simulink model "JABS"  (R2018b)
settings: Solver=FixedStepDiscrete  StartTime=0.0  StopTime=10.0  FixedStep=0.01  RelTol=1e-3
(part 1 of 2)
settings Model: Creator=gaohang  LastModifiedBy=gaohang
settings OptimizationCC: BlockReduction=off  DefaultParameterBehavior=Inlined  UseDivisionForNetSlopeComputation=on  UseFloatMulNetSlope=on  DefaultUnderspecifiedDataType=single  UseSpecifiedMinMax=on  InlineInvariantSignals=on  PassReuseOutputArgsAs=Individual arguments  ZeroExternalMemoryAtStartup=off  ZeroInternalMemoryAtStartup=off  LifeSpan=inf  OptimizeBlockOrder=speed  DifferentSizesBufferReuse=on
settings DebuggingCC: SignalInfNanChecking=error  ReadBeforeWriteMsg=EnableAllAsError  WriteAfterWriteMsg=EnableAllAsError  WriteAfterReadMsg=EnableAllAsError  IntegerOverflowMsg=error  ParameterTunabilityLossMsg=error  UniqueDataStoreMsg=error  NonBusSignalsTreatedAsBus=error  IntegerSaturationMsg=error
settings ModelReferenceCC: UpdateModelReferenceTargets=IfOutOfDate
settings SFSimCC: SFSimEcho=off  CompileTimeRecursionLimit=0  MATLABDynamicMemAlloc=off
settings RTWCC: SystemTargetFile=autosar.tlc  GenCodeOnly=on  TemplateMakefile=ert_default_tmf  Description=AUTOSAR  GenerateReport=on  BuildConfiguration=Faster Runs  IncludeHyperlinkInReport=on  LaunchReport=on  GenerateTraceInfo=on  GenerateTraceReport=on  GenerateTraceReportSl=on  GenerateTraceReportSf=on  GenerateTraceReportEml=on  GenerateCodeMetricsReport=on
settings CodeAppCC: ForceParamTrailComments=on  IgnoreCustomStorageClasses=off  OperatorAnnotations=on  SimulinkDataObjDesc=on  SFDataObjDesc=on  MATLABFcnDesc=on  InsertBlockDesc=on  StateflowObjectComments=on  EnableCustomComments=on  ReqsInCode=on
settings STFCustomTargetCC: TargetLangStandard=C99 (ISO)  UtilityFuncGeneration=Shared location  MultiwordLength=256  ParMdlRefBuildCompliant=on  CompOptLevelCompliant=on  IncludeMdlTerminateFcn=off  CombineOutputUpdateFcns=on  CombineSignalStateStructs=on  SuppressErrorStatus=on  ERTCustomFileBanners=on  SupportNonFinite=off  SupportComplex=off  SupportContinuousTime=off  SupportNonInlinedSFcns=off  RemoveResetFunc=on  ParenthesesLevel=Maximum  CastingMode=Standards  MATLABClassNameForMDSCustomization=Simulink.SoftwareTarget.ERTCustomization  AutosarCompliant=on  UseToolchainInfoCompliant=on  GenerateSharedConstants=off  LookupTableObjectStructAxisOrder=2,1,3,4,...  LUTObjectStructOrderEvenSpacing=Size,Table,Breakpoints  SystemTargetFile=autosar.tlc
settings ERTTargetCC: TargetLangStandard=C99 (ISO)  UtilityFuncGeneration=Shared location  ConcurrentExecutionCompliant=off  IncludeMdlTerminateFcn=off  CombineSignalStateStructs=on  SuppressErrorStatus=on  SupportNonFinite=off  SupportComplex=off  ParenthesesLevel=Maximum  CastingMode=Standards  ModelStepFunctionPrototypeControlCompliant=off  CPPClassGenCompliant=off  AutosarCompliant=on  GenerateSharedConstants=off  LookupTableObjectStructAxisOrder=2,1,3,4,...  LUTObjectStructOrderEvenSpacing=Size,Table,Breakpoints  GenerateASAP2=on  InlinedParameterPlacement=NonHierarchical  ERTCustomFileTemplate=example_file_process.tlc  EnableSignedLeftShifts=off  EnableSignedRightShifts=off

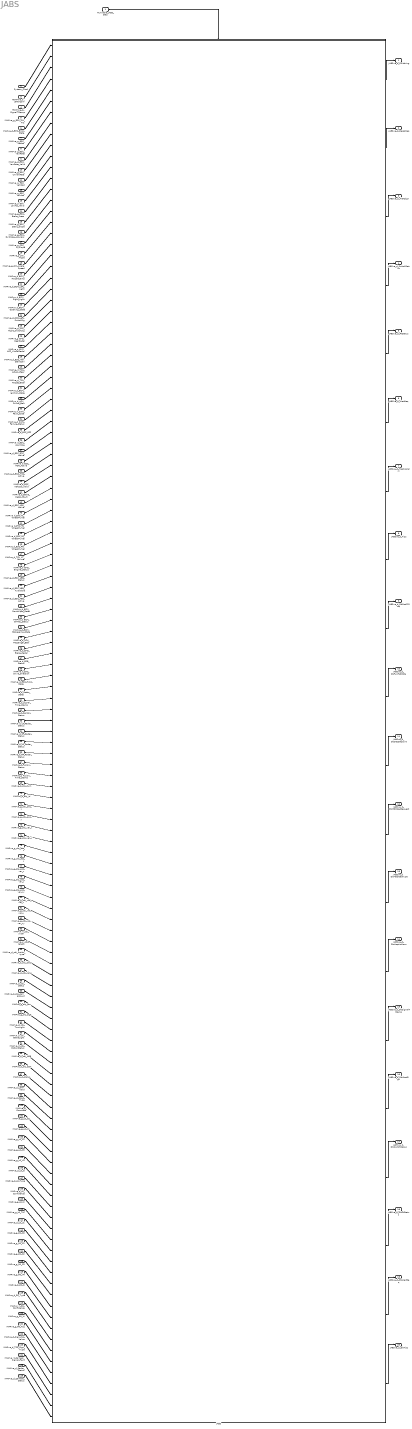
== system JABS ==
  Runnable_JABS_Step : Inport  SampleTime=0.01  OutputFunctionCall=on
  System_Clock : Inport  Port=2
  FDMMve_d_JaFcnConf : Inport  Port=3
  FDMMve_d_SignalTStamp : Inport  Port=4
  IMAPve_g_EPS_SW_Trq : Inport  Port=5
  IMAPve_d_EPS_Error_State : Inport  Port=6
  IMAPve_g_ESC_LatAcc : Inport  Port=7
  IMAPve_g_ESC_YawRate : Inport  Port=8
  IMAPve_d_ESC_YawRate_Valid : Inport  Port=9
  IMAPve_g_ESC_UnYawRate : Inport  Port=10
  IMAPve_g_ESC_VehSpd : Inport  Port=11
  IMAPve_g_ESC_LonAcc : Inport  Port=12
  IMAPve_d_ESC_LonAcc_Valid : Inport  Port=13
  IMAPve_g_ESC_Brake_Press : Inport  Port=14
  IMAPve_g_ESC_Static_Slope : Inport  Port=15
  IMAPve_g_ESC_DySlope_Accuracy : Inport  Port=16
  IMAPve_g_ESC_DySlope : Inport  Port=17
  IMAPve_g_SW_Angle : Inport  Port=18
  IMAPve_g_SW_Angle_Speed : Inport  Port=19
  IMAPve_d_BCM_HazardLamp : Inport  Port=20
  IMAPve_d_BCM_Left_Light : Inport  Port=21
  IMAPve_d_BCM_Right_Light : Inport  Port=22
  IMAPve_d_BCM_Opening_State : Inport  Port=23
  IMAPve_d_SCC_Left_SwitchSig : Inport  Port=24
  IMAPve_d_SCC_Right_SwitchSig : Inport  Port=25
  IMAPve_g_EMS_RealPedal : Inport  Port=26
  IMAPve_g_EMS_ACC_VirtualPedal : Inport  Port=27
  IMAPve_d_ESC_Veh_Standstill : Inport  Port=28
  IMAPve_d_TCU_Actual_Gear : Inport  Port=29
  IMAPve_d_TCU_Target_Gear : Inport  Port=30
  IMAPve_d_BCM_Ignition_State : Inport  Port=31
  IMAPve_d_ACU_Driver_Belt : Inport  Port=32
  IMAPve_d_SWS_Fault_Code : Inport  Port=33
  IMAPve_d_SWS_Failure_Status : Inport  Port=34
  IMAPve_d_ESC_OFF : Inport  Port=35
  IMAPve_d_ESC_AlarmSig : Inport  Port=36
  IMAPve_d_ESC_ESC_Active : Inport  Port=37
  IMAPve_d_ESC_MSR_Active : Inport  Port=38
  IMAPve_d_ESC_TCS_Active : Inport  Port=39
  IMAPve_d_ESC_VehSpd_Valid : Inport  Port=40
  IMAPve_d_Brake_Pedal_Fault : Inport  Port=41
  IMAPve_d_ESC_ABS_Active : Inport  Port=42
  IMAPve_d_ESC_FL_WheelPulVal : Inport  Port=43
  IMAPve_d_ESC_FR_WheelPulVal : Inport  Port=44
  IMAPve_d_ESC_RL_WheelPulVal : Inport  Port=45
  IMAPve_d_ESC_RR_WheelPulVal : Inport  Port=46
  IMAPve_d_TCU_AT_Failure : Inport  Port=47
  IMAPve_d_EMS_Engine_Status : Inport  Port=48
  IMAPve_d_ESC_AEB_Status : Inport  Port=49
  IMAPve_d_ESC_AEB_Available : Inport  Port=50
  IMAPve_d_ESC_AEB_Active : Inport  Port=51
  IMAPve_d_BCM_FrontWiper_State : Inport  Port=52
  IMAPve_d_BCM_CHMSL_Status : Inport  Port=53
  IMAPve_d_BCM_BrakeLamp_State : Inport  Port=54
  IMAPve_d_ACU_Passenger_Belt : Inport  Port=55
  IMAPve_d_EMS_Brake_Pedal : Inport  Port=56
  IMAPve_d_EPB_Status : Inport  Port=57
  IMAPve_d_ESC_Drive_Direction : Inport  Port=58
  IMAPve_d_ESC_Hold_State : Inport  Port=59
  IMAPve_d_Radar_State : Inport  Port=60
  IMAPve_d_Signal_Time_Stamp : Inport  Port=61
  IMAPve_d_Sensor_Status : Inport  Port=62
  IMAPve_d_LF_Radar_Status : Inport  Port=63
  IMAPve_d_RF_Radar_Status : Inport  Port=64
  IMAPve_d_LR_Radar_Status : Inport  Port=65
  IMAPve_d_RR_Radar_Status : Inport  Port=66
  IMAPve_d_Fusion_Status : Inport  Port=67
  IMAPve_g_Fusion_Time_Stamp : Inport  Port=68
  IMAPve_d_obj_Num : Inport  Port=69
  IMAPva_d_obj_id : Inport  Port=70
  IMAPva_g_obj_pos_x : Inport  Port=71
  IMAPva_g_obj_pos_y : Inport  Port=72
  IMAPva_g_obj_vel_x : Inport  Port=73
  IMAPva_g_obj_vel_y : Inport  Port=74
  IMAPva_g_obj_acc_x : Inport  Port=75
  IMAPva_g_obj_acc_y : Inport  Port=76
  IMAPva_g_obj_pos_var_x : Inport  Port=77
  IMAPva_g_obj_pos_var_y : Inport  Port=78
  IMAPva_g_obj_pos_var_xy : Inport  Port=79
  IMAPva_g_obj_vel_var_x : Inport  Port=80
  IMAPva_g_obj_vel_var_y : Inport  Port=81
  IMAPva_g_obj_vel_var_xy : Inport  Port=82
  IMAPva_g_obj_width : Inport  Port=83
  IMAPva_g_obj_length : Inport  Port=84
  IMAPva_d_obj_fusion_type : Inport  Port=85
  IMAPva_d_obj_class : Inport  Port=86
  IMAPva_d_obj_lane : Inport  Port=87
  IMAPva_d_obj_status : Inport  Port=88
  IMAPva_d_obj_cam_asso_id : Inport  Port=89
  IMAPva_g_obj_con : Inport  Port=90
  IMAPva_g_obj_age : Inport  Port=91
  IMAPva_d_obj_TurnLight : Inport  Port=92
  IMAPva_d_obj_BrakeLight : Inport  Port=93
  IMAPva_d_obj_MotionStatus : Inport  Port=94
  IMAPva_d_obj_AEB : Inport  Port=95
  IMAPva_d_obj_ESA : Inport  Port=96
  IMAPva_d_obj_JA : Inport  Port=97
  IMAPve_d_Lane_Valid : Inport  Port=98
  IMAPve_d_Road_Type : Inport  Port=99
  IMAPve_d_ConsArea : Inport  Port=100
  IMAPve_g_L0_C0 : Inport  Port=101
  IMAPve_g_L0_C1 : Inport  Port=102
  IMAPve_g_L0_C2 : Inport  Port=103
  IMAPve_g_L0_C3 : Inport  Port=104
  IMAPve_g_L0_VR : Inport  Port=105
  IMAPve_d_L0_Q : Inport  Port=106
  IMAPve_d_L0_Type : Inport  Port=107
  IMAPve_g_L0_Confidence : Inport  Port=108
  IMAPve_g_L0_W : Inport  Port=109
  IMAPve_g_L0_TLC : Inport  Port=110
  IMAPve_d_L0_LC : Inport  Port=111
  IMAPve_g_R0_C0 : Inport  Port=112
  IMAPve_g_R0_C1 : Inport  Port=113
  IMAPve_g_R0_C2 : Inport  Port=114
  IMAPve_g_R0_C3 : Inport  Port=115
  IMAPve_g_R0_VR : Inport  Port=116
  IMAPve_d_R0_Q : Inport  Port=117
  IMAPve_d_R0_Type : Inport  Port=118
  IMAPve_g_R0_Confidence : Inport  Port=119
  IMAPve_g_R0_W : Inport  Port=120
  IMAPve_g_R0_TLC : Inport  Port=121
  IMAPve_d_Sign_ISA_Value : Inport  Port=122
  IMAPve_d_TSR_Sign_Type : Inport  Port=123
  IMAPve_d_Camera_Signal_Fault : Inport  Port=124
  IMAPve_d_Radar_Status : Inport  Port=125
  IMAPve_d_Camera_Status : Inport  Port=126
  JABS : Subsystem  TreatAsAtomicUnit=on
  JABSve_d_Switching : Outport  OutDataTypeStr=UInt16
  JABSve_d_DecelReq : Outport  Port=2  OutDataTypeStr=T_M_Nm_Float32
  JABSve_d_AlertSign : Outport  Port=3  OutDataTypeStr=UInt16
  JABSve_d_SwitchStatus : Outport  Port=4  OutDataTypeStr=UInt16
  JABSve_d_FltStatus : Outport  Port=5  OutDataTypeStr=UInt16
  JABSve_d_AlertReq : Outport  Port=6  OutDataTypeStr=UInt16
  JABSve_d_HapticAlarm : Outport  Port=7  OutDataTypeStr=UInt16
  JABSve_d_Tips : Outport  Port=8  OutDataTypeStr=UInt16
  JABSve_d_DbPrefillReq : Outport  Port=9  OutDataTypeStr=UInt16
  JABSve_d_DbFunFARCSta : Outport  Port=10  OutDataTypeStr=UInt16
  JABSve_d_DbDecSetpoint : Outport  Port=11  OutDataTypeStr=T_M_Nm_Float32
  JABSve_d_DbMDDdecRequest : Outport  Port=12  OutDataTypeStr=UInt16
  JABSve_d_DbMDDdecType : Outport  Port=13  OutDataTypeStr=UInt16
  JABSve_d_DbHapticAlarm : Outport  Port=14  OutDataTypeStr=UInt16
  JABSve_d_DbSignalTStamp : Outport  Port=15  OutDataTypeStr=UInt16
  JABSve_d_DbAlertSign : Outport  Port=16  OutDataTypeStr=UInt16
  JABSve_d_DbSwitchStatus : Outport  Port=17  OutDataTypeStr=UInt16
  JABSve_d_DbFltStatus : Outport  Port=18  OutDataTypeStr=UInt16
  JABSve_d_DbAlertReq : Outport  Port=19  OutDataTypeStr=UInt16
  JABSve_d_DbTips : Outport  Port=20  OutDataTypeStr=UInt16
  wires:
  Runnable_JABS_Step/1 -> JABS/Trigger
  JABS/1(JABSve_d_Switching) -> JABSve_d_Switching/1
  JABS/2(JABSve_d_DecelReq) -> JABSve_d_DecelReq/1
  JABS/3(JABSve_d_AlertSign) -> JABSve_d_AlertSign/1
  JABS/4(JABSve_d_SwitchStatus) -> JABSve_d_SwitchStatus/1
  JABS/5(JABSve_d_FltStatus) -> JABSve_d_FltStatus/1
  JABS/6(JABSve_d_AlertReq) -> JABSve_d_AlertReq/1
  JABS/7(JABSve_d_HapticAlarm) -> JABSve_d_HapticAlarm/1
  JABS/8(JABSve_d_Tips) -> JABSve_d_Tips/1
  JABS/9(JABSve_d_DbPrefillReq) -> JABSve_d_DbPrefillReq/1
  JABS/10(JABSve_d_DbFunFARCSta) -> JABSve_d_DbFunFARCSta/1
  JABS/11(JABSve_d_DbDecSetpoint) -> JABSve_d_DbDecSetpoint/1
  JABS/12(JABSve_d_DbMDDdecRequest) -> JABSve_d_DbMDDdecRequest/1
  JABS/13(JABSve_d_DbMDDdecType) -> JABSve_d_DbMDDdecType/1
  JABS/14(JABSve_d_DbHapticAlarm) -> JABSve_d_DbHapticAlarm/1
  JABS/15(JABSve_d_DbSignalTStamp) -> JABSve_d_DbSignalTStamp/1
  JABS/16(JABSve_d_DbAlertSign) -> JABSve_d_DbAlertSign/1
  JABS/17(JABSve_d_DbSwitchStatus) -> JABSve_d_DbSwitchStatus/1
  JABS/18(JABSve_d_DbFltStatus) -> JABSve_d_DbFltStatus/1
  JABS/19(JABSve_d_DbAlertReq) -> JABSve_d_DbAlertReq/1
  JABS/20(JABSve_d_DbTips) -> JABSve_d_DbTips/1
  System_Clock/1 -> JABS/1(System_Clock)
  FDMMve_d_JaFcnConf/1 -> JABS/2(FDMMve_d_JaFcnConf)
  FDMMve_d_SignalTStamp/1 -> JABS/3(FDMMve_d_SignalTStamp)
  IMAPve_g_EPS_SW_Trq/1 -> JABS/4(IMAPve_g_EPS_SW_Trq)
  IMAPve_d_EPS_Error_State/1 -> JABS/5(IMAPve_d_EPS_Error_State)
  IMAPve_g_ESC_LatAcc/1 -> JABS/6(IMAPve_g_ESC_LatAcc)
  IMAPve_g_ESC_YawRate/1 -> JABS/7(IMAPve_g_ESC_YawRate)
  IMAPve_d_ESC_YawRate_Valid/1 -> JABS/8(IMAPve_d_ESC_YawRate_Valid)
  IMAPve_g_ESC_UnYawRate/1 -> JABS/9(IMAPve_g_ESC_UnYawRate)
  IMAPve_g_ESC_VehSpd/1 -> JABS/10(IMAPve_g_ESC_VehSpd)
  IMAPve_g_ESC_LonAcc/1 -> JABS/11(IMAPve_g_ESC_LonAcc)
  IMAPve_d_ESC_LonAcc_Valid/1 -> JABS/12(IMAPve_d_ESC_LonAcc_Valid)
  IMAPve_g_ESC_Brake_Press/1 -> JABS/13(IMAPve_g_ESC_Brake_Press)
  IMAPve_g_ESC_Static_Slope/1 -> JABS/14(IMAPve_g_ESC_Static_Slope)
  IMAPve_g_ESC_DySlope_Accuracy/1 -> JABS/15(IMAPve_g_ESC_DySlope_Accuracy)
  IMAPve_g_ESC_DySlope/1 -> JABS/16(IMAPve_g_ESC_DySlope)
  IMAPve_g_SW_Angle/1 -> JABS/17(IMAPve_g_SW_Angle)
  IMAPve_g_SW_Angle_Speed/1 -> JABS/18(IMAPve_g_SW_Angle_Speed)
  IMAPve_d_BCM_HazardLamp/1 -> JABS/19(IMAPve_d_BCM_HazardLamp)
  IMAPve_d_BCM_Left_Light/1 -> JABS/20(IMAPve_d_BCM_Left_Light)
  IMAPve_d_BCM_Right_Light/1 -> JABS/21(IMAPve_d_BCM_Right_Light)
  IMAPve_d_BCM_Opening_State/1 -> JABS/22(IMAPve_d_BCM_Opening_State)
  IMAPve_d_SCC_Left_SwitchSig/1 -> JABS/23(IMAPve_d_SCC_Left_SwitchSig)
  IMAPve_d_SCC_Right_SwitchSig/1 -> JABS/24(IMAPve_d_SCC_Right_SwitchSig)
  IMAPve_g_EMS_RealPedal/1 -> JABS/25(IMAPve_g_EMS_RealPedal)
  IMAPve_g_EMS_ACC_VirtualPedal/1 -> JABS/26(IMAPve_g_EMS_ACC_VirtualPedal)
  IMAPve_d_ESC_Veh_Standstill/1 -> JABS/27(IMAPve_d_ESC_Veh_Standstill)
  IMAPve_d_TCU_Actual_Gear/1 -> JABS/28(IMAPve_d_TCU_Actual_Gear)
  IMAPve_d_TCU_Target_Gear/1 -> JABS/29(IMAPve_d_TCU_Target_Gear)
  IMAPve_d_BCM_Ignition_State/1 -> JABS/30(IMAPve_d_BCM_Ignition_State)
  IMAPve_d_ACU_Driver_Belt/1 -> JABS/31(IMAPve_d_ACU_Driver_Belt)
  IMAPve_d_SWS_Fault_Code/1 -> JABS/32(IMAPve_d_SWS_Fault_Code)
  IMAPve_d_SWS_Failure_Status/1 -> JABS/33(IMAPve_d_SWS_Failure_Status)
  IMAPve_d_ESC_OFF/1 -> JABS/34(IMAPve_d_ESC_OFF)
  IMAPve_d_ESC_AlarmSig/1 -> JABS/35(IMAPve_d_ESC_AlarmSig)
  IMAPve_d_ESC_ESC_Active/1 -> JABS/36(IMAPve_d_ESC_ESC_Active)
  IMAPve_d_ESC_MSR_Active/1 -> JABS/37(IMAPve_d_ESC_MSR_Active)
  IMAPve_d_ESC_TCS_Active/1 -> JABS/38(IMAPve_d_ESC_TCS_Active)
  IMAPve_d_ESC_VehSpd_Valid/1 -> JABS/39(IMAPve_d_ESC_VehSpd_Valid)
  IMAPve_d_Brake_Pedal_Fault/1 -> JABS/40(IMAPve_d_Brake_Pedal_Fault)
  IMAPve_d_ESC_ABS_Active/1 -> JABS/41(IMAPve_d_ESC_ABS_Active)
  IMAPve_d_ESC_FL_WheelPulVal/1 -> JABS/42(IMAPve_d_ESC_FL_WheelPulVal)
  IMAPve_d_ESC_FR_WheelPulVal/1 -> JABS/43(IMAPve_d_ESC_FR_WheelPulVal)
  IMAPve_d_ESC_RL_WheelPulVal/1 -> JABS/44(IMAPve_d_ESC_RL_WheelPulVal)
  IMAPve_d_ESC_RR_WheelPulVal/1 -> JABS/45(IMAPve_d_ESC_RR_WheelPulVal)
  IMAPve_d_TCU_AT_Failure/1 -> JABS/46(IMAPve_d_TCU_AT_Failure)
  IMAPve_d_EMS_Engine_Status/1 -> JABS/47(IMAPve_d_EMS_Engine_Status)
  IMAPve_d_ESC_AEB_Status/1 -> JABS/48(IMAPve_d_ESC_AEB_Status)
  IMAPve_d_ESC_AEB_Available/1 -> JABS/49(IMAPve_d_ESC_AEB_Available)
  IMAPve_d_ESC_AEB_Active/1 -> JABS/50(IMAPve_d_ESC_AEB_Active)
  IMAPve_d_BCM_FrontWiper_State/1 -> JABS/51(IMAPve_d_BCM_FrontWiper_State)
  IMAPve_d_BCM_CHMSL_Status/1 -> JABS/52(IMAPve_d_BCM_CHMSL_Status)
  IMAPve_d_BCM_BrakeLamp_State/1 -> JABS/53(IMAPve_d_BCM_BrakeLamp_State)
  IMAPve_d_ACU_Passenger_Belt/1 -> JABS/54(IMAPve_d_ACU_Passenger_Belt)
  IMAPve_d_EMS_Brake_Pedal/1 -> JABS/55(IMAPve_d_EMS_Brake_Pedal)
  IMAPve_d_EPB_Status/1 -> JABS/56(IMAPve_d_EPB_Status)
  IMAPve_d_ESC_Drive_Direction/1 -> JABS/57(IMAPve_d_ESC_Drive_Direction)
  IMAPve_d_ESC_Hold_State/1 -> JABS/58(IMAPve_d_ESC_Hold_State)
  IMAPve_d_Radar_State/1 -> JABS/59(IMAPve_d_Radar_State)
  IMAPve_d_Signal_Time_Stamp/1 -> JABS/60(IMAPve_d_Signal_Time_Stamp)
  IMAPve_d_Sensor_Status/1 -> JABS/61(IMAPve_d_Sensor_Status)
  IMAPve_d_LF_Radar_Status/1 -> JABS/62(IMAPve_d_LF_Radar_Status)
  IMAPve_d_RF_Radar_Status/1 -> JABS/63(IMAPve_d_RF_Radar_Status)
  IMAPve_d_LR_Radar_Status/1 -> JABS/64(IMAPve_d_LR_Radar_Status)
  IMAPve_d_RR_Radar_Status/1 -> JABS/65(IMAPve_d_RR_Radar_Status)
  IMAPve_d_Fusion_Status/1 -> JABS/66(IMAPve_d_Fusion_Status)
  IMAPve_g_Fusion_Time_Stamp/1 -> JABS/67(IMAPve_g_Fusion_Time_Stamp)
  IMAPve_d_obj_Num/1 -> JABS/68(IMAPve_d_obj_Num)
  IMAPva_d_obj_id/1 -> JABS/69(IMAPva_d_obj_id)
  IMAPva_g_obj_pos_x/1 -> JABS/70(IMAPva_g_obj_pos_x)
  IMAPva_g_obj_pos_y/1 -> JABS/71(IMAPva_g_obj_pos_y)
  IMAPva_g_obj_vel_x/1 -> JABS/72(IMAPva_g_obj_vel_x)
  IMAPva_g_obj_vel_y/1 -> JABS/73(IMAPva_g_obj_vel_y)
  IMAPva_g_obj_acc_x/1 -> JABS/74(IMAPva_g_obj_acc_x)
  IMAPva_g_obj_acc_y/1 -> JABS/75(IMAPva_g_obj_acc_y)
  IMAPva_g_obj_pos_var_x/1 -> JABS/76(IMAPva_g_obj_pos_var_x)
  IMAPva_g_obj_pos_var_y/1 -> JABS/77(IMAPva_g_obj_pos_var_y)
  IMAPva_g_obj_pos_var_xy/1 -> JABS/78(IMAPva_g_obj_pos_var_xy)
  IMAPva_g_obj_vel_var_x/1 -> JABS/79(IMAPva_g_obj_vel_var_x)
  IMAPva_g_obj_vel_var_y/1 -> JABS/80(IMAPva_g_obj_vel_var_y)
  IMAPva_g_obj_vel_var_xy/1 -> JABS/81(IMAPva_g_obj_vel_var_xy)
  IMAPva_g_obj_width/1 -> JABS/82(IMAPva_g_obj_width)
  IMAPva_g_obj_length/1 -> JABS/83(IMAPva_g_obj_length)
  IMAPva_d_obj_fusion_type/1 -> JABS/84(IMAPva_d_obj_fusion_type)
  IMAPva_d_obj_class/1 -> JABS/85(IMAPva_d_obj_class)
  IMAPva_d_obj_lane/1 -> JABS/86(IMAPva_d_obj_lane)
  IMAPva_d_obj_status/1 -> JABS/87(IMAPva_d_obj_status)
  IMAPva_d_obj_cam_asso_id/1 -> JABS/88(IMAPva_d_obj_cam_asso_id)
  IMAPva_g_obj_con/1 -> JABS/89(IMAPva_g_obj_con)
  IMAPva_g_obj_age/1 -> JABS/90(IMAPva_g_obj_age)
  IMAPva_d_obj_TurnLight/1 -> JABS/91(IMAPva_d_obj_TurnLight)
  IMAPva_d_obj_BrakeLight/1 -> JABS/92(IMAPva_d_obj_BrakeLight)
  IMAPva_d_obj_MotionStatus/1 -> JABS/93(IMAPva_d_obj_MotionStatus)
  IMAPva_d_obj_AEB/1 -> JABS/94(IMAPva_d_obj_AEB)
  IMAPva_d_obj_ESA/1 -> JABS/95(IMAPva_d_obj_ESA)
  IMAPva_d_obj_JA/1 -> JABS/96(IMAPva_d_obj_JA)
  IMAPve_d_Lane_Valid/1 -> JABS/97(IMAPve_d_Lane_Valid)
  IMAPve_d_Road_Type/1 -> JABS/98(IMAPve_d_Road_Type)
  IMAPve_d_ConsArea/1 -> JABS/99(IMAPve_d_ConsArea)
  IMAPve_g_L0_C0/1 -> JABS/100(IMAPve_g_L0_C0)
  IMAPve_g_L0_C1/1 -> JABS/101(IMAPve_g_L0_C1)
  IMAPve_g_L0_C2/1 -> JABS/102(IMAPve_g_L0_C2)
  IMAPve_g_L0_C3/1 -> JABS/103(IMAPve_g_L0_C3)
  IMAPve_g_L0_VR/1 -> JABS/104(IMAPve_g_L0_VR)
  IMAPve_d_L0_Q/1 -> JABS/105(IMAPve_d_L0_Q)
  IMAPve_d_L0_Type/1 -> JABS/106(IMAPve_d_L0_Type)
  IMAPve_g_L0_Confidence/1 -> JABS/107(IMAPve_g_L0_Confidence)
  IMAPve_g_L0_W/1 -> JABS/108(IMAPve_g_L0_W)
  IMAPve_g_L0_TLC/1 -> JABS/109(IMAPve_g_L0_TLC)
  IMAPve_d_L0_LC/1 -> JABS/110(IMAPve_d_L0_LC)
  IMAPve_g_R0_C0/1 -> JABS/111(IMAPve_g_R0_C0)
  IMAPve_g_R0_C1/1 -> JABS/112(IMAPve_g_R0_C1)
  IMAPve_g_R0_C2/1 -> JABS/113(IMAPve_g_R0_C2)
  IMAPve_g_R0_C3/1 -> JABS/114(IMAPve_g_R0_C3)
  IMAPve_g_R0_VR/1 -> JABS/115(IMAPve_g_R0_VR)
  IMAPve_d_R0_Q/1 -> JABS/116(IMAPve_d_R0_Q)
  IMAPve_d_R0_Type/1 -> JABS/117(IMAPve_d_R0_Type)
  IMAPve_g_R0_Confidence/1 -> JABS/118(IMAPve_g_R0_Confidence)
  IMAPve_g_R0_W/1 -> JABS/119(IMAPve_g_R0_W)
  IMAPve_g_R0_TLC/1 -> JABS/120(IMAPve_g_R0_TLC)
  IMAPve_d_Sign_ISA_Value/1 -> JABS/121(IMAPve_d_Sign_ISA_Value)
  IMAPve_d_TSR_Sign_Type/1 -> JABS/122(IMAPve_d_TSR_Sign_Type)
  IMAPve_d_Camera_Signal_Fault/1 -> JABS/123(IMAPve_d_Camera_Signal_Fault)
  IMAPve_d_Radar_Status/1 -> JABS/124(IMAPve_d_Radar_Status)
  IMAPve_d_Camera_Status/1 -> JABS/125(IMAPve_d_Camera_Status)

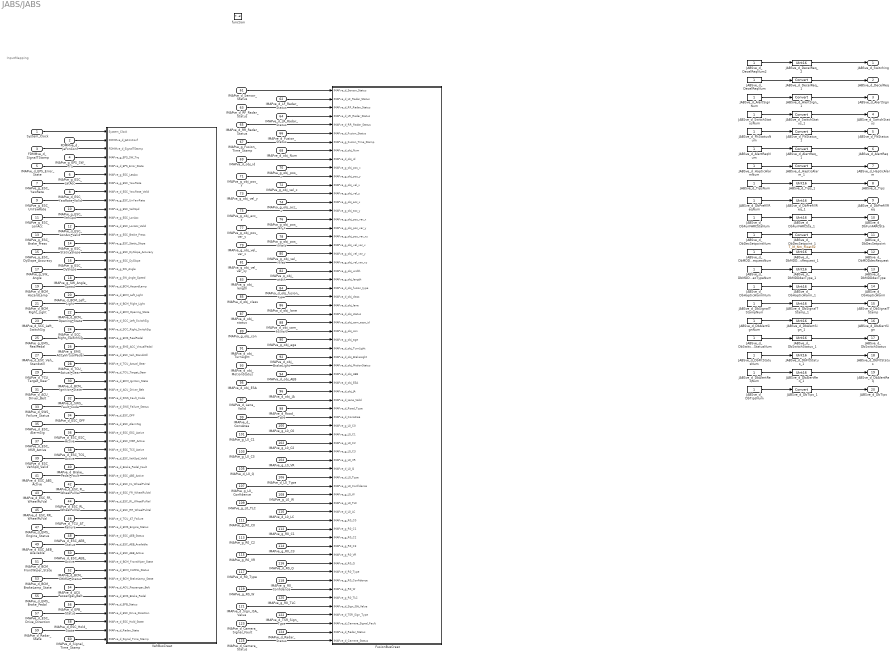
== system JABS/JABS ==
  note: InputMapping
  System_Clock : Inport
  FDMMve_d_JaFcnConf : Inport  Port=2
  FDMMve_d_SignalTStamp : Inport  Port=3
  IMAPve_g_EPS_SW_Trq : Inport  Port=4
  IMAPve_d_EPS_Error_State : Inport  Port=5
  IMAPve_g_ESC_LatAcc : Inport  Port=6
  IMAPve_g_ESC_YawRate : Inport  Port=7
  IMAPve_d_ESC_YawRate_Valid : Inport  Port=8
  IMAPve_g_ESC_UnYawRate : Inport  Port=9
  IMAPve_g_ESC_VehSpd : Inport  Port=10
  IMAPve_g_ESC_LonAcc : Inport  Port=11
  IMAPve_d_ESC_LonAcc_Valid : Inport  Port=12
  IMAPve_g_ESC_Brake_Press : Inport  Port=13
  IMAPve_g_ESC_Static_Slope : Inport  Port=14
  IMAPve_g_ESC_DySlope_Accuracy : Inport  Port=15
  IMAPve_g_ESC_DySlope : Inport  Port=16
  IMAPve_g_SW_Angle : Inport  Port=17
  IMAPve_g_SW_Angle_Speed : Inport  Port=18
  IMAPve_d_BCM_HazardLamp : Inport  Port=19
  IMAPve_d_BCM_Left_Light : Inport  Port=20
  IMAPve_d_BCM_Right_Light : Inport  Port=21
  IMAPve_d_BCM_Opening_State : Inport  Port=22
  IMAPve_d_SCC_Left_SwitchSig : Inport  Port=23
  IMAPve_d_SCC_Right_SwitchSig : Inport  Port=24
  IMAPve_g_EMS_RealPedal : Inport  Port=25
  IMAPve_g_EMS_ACC_VirtualPedal : Inport  Port=26
  IMAPve_d_ESC_Veh_Standstill : Inport  Port=27
  IMAPve_d_TCU_Actual_Gear : Inport  Port=28
  IMAPve_d_TCU_Target_Gear : Inport  Port=29
  IMAPve_d_BCM_Ignition_State : Inport  Port=30
  IMAPve_d_ACU_Driver_Belt : Inport  Port=31
  IMAPve_d_SWS_Fault_Code : Inport  Port=32
  IMAPve_d_SWS_Failure_Status : Inport  Port=33
  IMAPve_d_ESC_OFF : Inport  Port=34
  IMAPve_d_ESC_AlarmSig : Inport  Port=35
  IMAPve_d_ESC_ESC_Active : Inport  Port=36
  IMAPve_d_ESC_MSR_Active : Inport  Port=37
  IMAPve_d_ESC_TCS_Active : Inport  Port=38
  IMAPve_d_ESC_VehSpd_Valid : Inport  Port=39
  IMAPve_d_Brake_Pedal_Fault : Inport  Port=40
  IMAPve_d_ESC_ABS_Active : Inport  Port=41
  IMAPve_d_ESC_FL_WheelPulVal : Inport  Port=42
  IMAPve_d_ESC_FR_WheelPulVal : Inport  Port=43
  IMAPve_d_ESC_RL_WheelPulVal : Inport  Port=44
  IMAPve_d_ESC_RR_WheelPulVal : Inport  Port=45
  IMAPve_d_TCU_AT_Failure : Inport  Port=46
  IMAPve_d_EMS_Engine_Status : Inport  Port=47
  IMAPve_d_ESC_AEB_Status : Inport  Port=48
  IMAPve_d_ESC_AEB_Available : Inport  Port=49
  IMAPve_d_ESC_AEB_Active : Inport  Port=50
  IMAPve_d_BCM_FrontWiper_State : Inport  Port=51
  IMAPve_d_BCM_CHMSL_Status : Inport  Port=52
  IMAPve_d_BCM_BrakeLamp_State : Inport  Port=53
  IMAPve_d_ACU_Passenger_Belt : Inport  Port=54
  IMAPve_d_EMS_Brake_Pedal : Inport  Port=55
  IMAPve_d_EPB_Status : Inport  Port=56
  IMAPve_d_ESC_Drive_Direction : Inport  Port=57
  IMAPve_d_ESC_Hold_State : Inport  Port=58
  IMAPve_d_Radar_State : Inport  Port=59
  IMAPve_d_Signal_Time_Stamp : Inport  Port=60
  IMAPve_d_Sensor_Status : Inport  Port=61
  IMAPve_d_LF_Radar_Status : Inport  Port=62
  IMAPve_d_RF_Radar_Status : Inport  Port=63
  IMAPve_d_LR_Radar_Status : Inport  Port=64
  IMAPve_d_RR_Radar_Status : Inport  Port=65
  IMAPve_d_Fusion_Status : Inport  Port=66
  IMAPve_g_Fusion_Time_Stamp : Inport  Port=67
  IMAPve_d_obj_Num : Inport  Port=68
  IMAPva_d_obj_id : Inport  Port=69
  IMAPva_g_obj_pos_x : Inport  Port=70
  IMAPva_g_obj_pos_y : Inport  Port=71
  IMAPva_g_obj_vel_x : Inport  Port=72
  IMAPva_g_obj_vel_y : Inport  Port=73
  IMAPva_g_obj_acc_x : Inport  Port=74
  IMAPva_g_obj_acc_y : Inport  Port=75
  IMAPva_g_obj_pos_var_x : Inport  Port=76
  IMAPva_g_obj_pos_var_y : Inport  Port=77
  IMAPva_g_obj_pos_var_xy : Inport  Port=78
  IMAPva_g_obj_vel_var_x : Inport  Port=79
  IMAPva_g_obj_vel_var_y : Inport  Port=80
  IMAPva_g_obj_vel_var_xy : Inport  Port=81
  IMAPva_g_obj_width : Inport  Port=82
  IMAPva_g_obj_length : Inport  Port=83
  IMAPva_d_obj_fusion_type : Inport  Port=84
  IMAPva_d_obj_class : Inport  Port=85
  IMAPva_d_obj_lane : Inport  Port=86
  IMAPva_d_obj_status : Inport  Port=87
  IMAPva_d_obj_cam_asso_id : Inport  Port=88
  IMAPva_g_obj_con : Inport  Port=89
  IMAPva_g_obj_age : Inport  Port=90
  IMAPva_d_obj_TurnLight : Inport  Port=91
  IMAPva_d_obj_BrakeLight : Inport  Port=92
  IMAPva_d_obj_MotionStatus : Inport  Port=93
  IMAPva_d_obj_AEB : Inport  Port=94
  IMAPva_d_obj_ESA : Inport  Port=95
  IMAPva_d_obj_JA : Inport  Port=96
  IMAPve_d_Lane_Valid : Inport  Port=97
  IMAPve_d_Road_Type : Inport  Port=98
  IMAPve_d_ConsArea : Inport  Port=99
  IMAPve_g_L0_C0 : Inport  Port=100
  IMAPve_g_L0_C1 : Inport  Port=101
  IMAPve_g_L0_C2 : Inport  Port=102
  IMAPve_g_L0_C3 : Inport  Port=103
  IMAPve_g_L0_VR : Inport  Port=104
  IMAPve_d_L0_Q : Inport  Port=105
  IMAPve_d_L0_Type : Inport  Port=106
  IMAPve_g_L0_Confidence : Inport  Port=107
  IMAPve_g_L0_W : Inport  Port=108
  IMAPve_g_L0_TLC : Inport  Port=109
  IMAPve_d_L0_LC : Inport  Port=110
  IMAPve_g_R0_C0 : Inport  Port=111
  IMAPve_g_R0_C1 : Inport  Port=112
  IMAPve_g_R0_C2 : Inport  Port=113
  IMAPve_g_R0_C3 : Inport  Port=114
  IMAPve_g_R0_VR : Inport  Port=115
  IMAPve_d_R0_Q : Inport  Port=116
  IMAPve_d_R0_Type : Inport  Port=117
  IMAPve_g_R0_Confidence : Inport  Port=118
  IMAPve_g_R0_W : Inport  Port=119
  IMAPve_g_R0_TLC : Inport  Port=120
  IMAPve_d_Sign_ISA_Value : Inport  Port=121
  IMAPve_d_TSR_Sign_Type : Inport  Port=122
  IMAPve_d_Camera_Signal_Fault : Inport  Port=123
  IMAPve_d_Radar_Status : Inport  Port=124
  IMAPve_d_Camera_Status : Inport  Port=125
  function : TriggerPort  TriggerType=function-call  VariantControl=Variant  SampleTimeType=periodic  SampleTime=-1
  FusionBusCreat : Subsystem
  JABSve_d_AlertReqNum : Constant  OutDataTypeStr=uint8
  JABSve_d_AlertReq_1 : DataTypeConversion
  JABSve_d_AlertSignNum : Constant  OutDataTypeStr=uint8  SampleTime=-1
  JABSve_d_AlertSign_1 : DataTypeConversion
  JABSve_d_DbAlertReqNum : Constant  OutDataTypeStr=uint8
  JABSve_d_DbAlertReq_1 : DataTypeConversion  OutDataTypeStr=UInt16
  JABSve_d_DbAlertSignNum : Constant  OutDataTypeStr=uint8
  JABSve_d_DbAlertSign_1 : DataTypeConversion  OutDataTypeStr=UInt16
  JABSve_d_DbDecSetpointNum : Constant  OutDataTypeStr=uint8
  JABSve_d_DbDecSetpoint_1 : DataTypeConversion  OutDataTypeStr=T_M_Nm_Float32
  JABSve_d_DbFltStatusNum : Constant  OutDataTypeStr=uint8
  JABSve_d_DbFltStatus_1 : DataTypeConversion  OutDataTypeStr=UInt16
  JABSve_d_DbFunFARCStaNum : Constant  OutDataTypeStr=uint8
  JABSve_d_DbFunFARCSta_1 : DataTypeConversion  OutDataTypeStr=UInt16
  JABSve_d_DbHapticAlarmNum : Constant  OutDataTypeStr=uint8
  JABSve_d_DbHapticAlarm_1 : DataTypeConversion  OutDataTypeStr=UInt16
  JABSve_d_DbMDDdecRequestNum : Constant  OutDataTypeStr=uint8
  JABSve_d_DbMDDdecRequest_1 : DataTypeConversion  OutDataTypeStr=UInt16
  JABSve_d_DbMDDdecTypeNum : Constant  OutDataTypeStr=uint8
  JABSve_d_DbMDDdecType_1 : DataTypeConversion  OutDataTypeStr=UInt16
  JABSve_d_DbPrefillReqNum : Constant  OutDataTypeStr=uint8
  JABSve_d_DbPrefillReq_1 : DataTypeConversion  OutDataTypeStr=UInt16
  JABSve_d_DbSignalTStampNum : Constant  OutDataTypeStr=uint8
  JABSve_d_DbSignalTStamp_1 : DataTypeConversion  OutDataTypeStr=UInt16
  JABSve_d_DbSwitchStatusNum : Constant  OutDataTypeStr=uint8
  JABSve_d_DbSwitchStatus_1 : DataTypeConversion  OutDataTypeStr=UInt16
  JABSve_d_DbTipsNum : Constant  OutDataTypeStr=uint8
  JABSve_d_DbTips_1 : DataTypeConversion
  JABSve_d_DecelReqNum : Constant  OutDataTypeStr=uint8
  JABSve_d_DecelReqNum2 : Constant  OutDataTypeStr=uint8
  JABSve_d_DecelReq_1 : DataTypeConversion
  JABSve_d_DecelReq_2 : DataTypeConversion  OutDataTypeStr=UInt16
  JABSve_d_FltStatusNum : Constant  OutDataTypeStr=uint8
  JABSve_d_FltStatus_1 : DataTypeConversion
  JABSve_d_HapticAlarmNum : Constant  OutDataTypeStr=uint8
  JABSve_d_HapticAlarm_1 : DataTypeConversion
  JABSve_d_SwitchStatusNum : Constant  OutDataTypeStr=uint8  SampleTime=-1
  JABSve_d_SwitchStatus_1 : DataTypeConversion
  JABSve_d_TipsNum : Constant  OutDataTypeStr=uint8
  JABSve_d_Tips_1 : DataTypeConversion  OutDataTypeStr=UInt16
  VehBusCreat : Subsystem
  JABSve_d_Switching : Outport  OutDataTypeStr=UInt16
  JABSve_d_DecelReq : Outport  Port=2  OutDataTypeStr=T_M_Nm_Float32
  JABSve_d_AlertSign : Outport  Port=3  OutDataTypeStr=UInt16
  JABSve_d_SwitchStatus : Outport  Port=4  OutDataTypeStr=UInt16
  JABSve_d_FltStatus : Outport  Port=5  OutDataTypeStr=UInt16
  JABSve_d_AlertReq : Outport  Port=6  OutDataTypeStr=UInt16
  JABSve_d_HapticAlarm : Outport  Port=7  OutDataTypeStr=UInt16
  JABSve_d_Tips : Outport  Port=8  OutDataTypeStr=UInt16
  JABSve_d_DbPrefillReq : Outport  Port=9  OutDataTypeStr=UInt16
  JABSve_d_DbFunFARCSta : Outport  Port=10  OutDataTypeStr=UInt16
  JABSve_d_DbDecSetpoint : Outport  Port=11  OutDataTypeStr=T_M_Nm_Float32
  JABSve_d_DbMDDdecRequest : Outport  Port=12  OutDataTypeStr=UInt16
  JABSve_d_DbMDDdecType : Outport  Port=13  OutDataTypeStr=UInt16
  JABSve_d_DbHapticAlarm : Outport  Port=14  OutDataTypeStr=UInt16
  JABSve_d_DbSignalTStamp : Outport  Port=15  OutDataTypeStr=UInt16
  JABSve_d_DbAlertSign : Outport  Port=16  OutDataTypeStr=UInt16
  JABSve_d_DbSwitchStatus : Outport  Port=17  OutDataTypeStr=UInt16
  JABSve_d_DbFltStatus : Outport  Port=18  OutDataTypeStr=UInt16
  JABSve_d_DbAlertReq : Outport  Port=19  OutDataTypeStr=UInt16
  JABSve_d_DbTips : Outport  Port=20  OutDataTypeStr=UInt16
  wires:
  JABSve_d_DecelReqNum2/1 -> JABSve_d_DecelReq_2/1
  JABSve_d_DecelReqNum/1 -> JABSve_d_DecelReq_1/1
  JABSve_d_DecelReq_1/1 -> JABSve_d_DecelReq/1
  JABSve_d_AlertSignNum/1 -> JABSve_d_AlertSign_1/1
  JABSve_d_AlertSign_1/1 -> JABSve_d_AlertSign/1
  JABSve_d_SwitchStatusNum/1 -> JABSve_d_SwitchStatus_1/1
  JABSve_d_SwitchStatus_1/1 -> JABSve_d_SwitchStatus/1
  JABSve_d_FltStatusNum/1 -> JABSve_d_FltStatus_1/1
  JABSve_d_FltStatus_1/1 -> JABSve_d_FltStatus/1
  JABSve_d_AlertReqNum/1 -> JABSve_d_AlertReq_1/1
  JABSve_d_AlertReq_1/1 -> JABSve_d_AlertReq/1
  JABSve_d_HapticAlarmNum/1 -> JABSve_d_HapticAlarm_1/1
  JABSve_d_HapticAlarm_1/1 -> JABSve_d_HapticAlarm/1
  JABSve_d_TipsNum/1 -> JABSve_d_Tips_1/1
  JABSve_d_Tips_1/1 -> JABSve_d_Tips/1
  JABSve_d_DbPrefillReqNum/1 -> JABSve_d_DbPrefillReq_1/1
  JABSve_d_DbPrefillReq_1/1 -> JABSve_d_DbPrefillReq/1
  JABSve_d_DbFunFARCStaNum/1 -> JABSve_d_DbFunFARCSta_1/1
  JABSve_d_DbFunFARCSta_1/1 -> JABSve_d_DbFunFARCSta/1
  JABSve_d_DbDecSetpointNum/1 -> JABSve_d_DbDecSetpoint_1/1
  JABSve_d_DbDecSetpoint_1/1 -> JABSve_d_DbDecSetpoint/1
  JABSve_d_DbMDDdecRequestNum/1 -> JABSve_d_DbMDDdecRequest_1/1
  JABSve_d_DbMDDdecRequest_1/1 -> JABSve_d_DbMDDdecRequest/1
  JABSve_d_DbMDDdecTypeNum/1 -> JABSve_d_DbMDDdecType_1/1
  JABSve_d_DbMDDdecType_1/1 -> JABSve_d_DbMDDdecType/1
  JABSve_d_DbHapticAlarmNum/1 -> JABSve_d_DbHapticAlarm_1/1
  JABSve_d_DbHapticAlarm_1/1 -> JABSve_d_DbHapticAlarm/1
  JABSve_d_DbSignalTStampNum/1 -> JABSve_d_DbSignalTStamp_1/1
  JABSve_d_DbSignalTStamp_1/1 -> JABSve_d_DbSignalTStamp/1
  JABSve_d_DbAlertSignNum/1 -> JABSve_d_DbAlertSign_1/1
  JABSve_d_DbAlertSign_1/1 -> JABSve_d_DbAlertSign/1
  JABSve_d_DbSwitchStatusNum/1 -> JABSve_d_DbSwitchStatus_1/1
  JABSve_d_DbSwitchStatus_1/1 -> JABSve_d_DbSwitchStatus/1
  JABSve_d_DbFltStatusNum/1 -> JABSve_d_DbFltStatus_1/1
  JABSve_d_DbFltStatus_1/1 -> JABSve_d_DbFltStatus/1
  JABSve_d_DbAlertReqNum/1 -> JABSve_d_DbAlertReq_1/1
  JABSve_d_DbAlertReq_1/1 -> JABSve_d_DbAlertReq/1
  JABSve_d_DbTipsNum/1 -> JABSve_d_DbTips_1/1
  JABSve_d_DbTips_1/1 -> JABSve_d_DbTips/1
  IMAPve_g_Fusion_Time_Stamp/1 -> FusionBusCreat/7(IMAPve_g_Fusion_Time_Stamp)
  FDMMve_d_SignalTStamp/1 -> VehBusCreat/3(FDMMve_d_SignalTStamp)
  IMAPve_d_RF_Radar_Status/1 -> FusionBusCreat/3(IMAPve_d_RF_Radar_Status)
  System_Clock/1 -> VehBusCreat/1(System_Clock)
  IMAPve_g_R0_Confidence/1 -> FusionBusCreat/58(IMAPve_g_R0_Confidence)
  IMAPve_d_Camera_Status/1 -> FusionBusCreat/65(IMAPve_d_Camera_Status)
  IMAPve_g_L0_C0/1 -> FusionBusCreat/40(IMAPve_g_L0_C0)
  IMAPve_g_ESC_UnYawRate/1 -> VehBusCreat/9(IMAPve_g_ESC_UnYawRate)
  IMAPve_d_Road_Type/1 -> FusionBusCreat/38(IMAPve_d_Road_Type)
  IMAPve_d_BCM_HazardLamp/1 -> VehBusCreat/19(IMAPve_d_BCM_HazardLamp)
  IMAPve_g_L0_C2/1 -> FusionBusCreat/42(IMAPve_g_L0_C2)
  IMAPve_d_ESC_YawRate_Valid/1 -> VehBusCreat/8(IMAPve_d_ESC_YawRate_Valid)
  IMAPve_d_Radar_Status/1 -> FusionBusCreat/64(IMAPve_d_Radar_Status)
  IMAPve_d_Camera_Signal_Fault/1 -> FusionBusCreat/63(IMAPve_d_Camera_Signal_Fault)
  IMAPva_g_obj_vel_var_y/1 -> FusionBusCreat/20(IMAPva_g_obj_vel_var_y)
  IMAPve_d_L0_Q/1 -> FusionBusCreat/45(IMAPve_d_L0_Q)
  IMAPve_d_TSR_Sign_Type/1 -> FusionBusCreat/62(IMAPve_d_TSR_Sign_Type)
  IMAPve_d_ESC_AEB_Active/1 -> VehBusCreat/50(IMAPve_d_ESC_AEB_Active)
  IMAPve_g_R0_VR/1 -> FusionBusCreat/55(IMAPve_g_R0_VR)
  IMAPva_g_obj_pos_y/1 -> FusionBusCreat/11(IMAPva_g_obj_pos_y)
  IMAPve_d_Sign_ISA_Value/1 -> FusionBusCreat/61(IMAPve_d_Sign_ISA_Value)
  IMAPve_g_ESC_LonAcc/1 -> VehBusCreat/11(IMAPve_g_ESC_LonAcc)
  IMAPve_g_L0_C1/1 -> FusionBusCreat/41(IMAPve_g_L0_C1)
  IMAPve_g_R0_TLC/1 -> FusionBusCreat/60(IMAPve_g_R0_TLC)
  IMAPva_d_obj_BrakeLight/1 -> FusionBusCreat/32(IMAPva_d_obj_BrakeLight)
  IMAPva_d_obj_ESA/1 -> FusionBusCreat/35(IMAPva_d_obj_ESA)
  IMAPve_d_ConsArea/1 -> FusionBusCreat/39(IMAPve_d_ConsArea)
  IMAPva_d_obj_id/1 -> FusionBusCreat/9(IMAPva_d_obj_id)
  IMAPve_d_ESC_Drive_Direction/1 -> VehBusCreat/57(IMAPve_d_ESC_Drive_Direction)
  IMAPve_g_L0_Confidence/1 -> FusionBusCreat/47(IMAPve_g_L0_Confidence)
  IMAPve_d_obj_Num/1 -> FusionBusCreat/8(IMAPve_d_obj_Num)
  IMAPve_g_R0_C2/1 -> FusionBusCreat/53(IMAPve_g_R0_C2)
  IMAPve_g_SW_Angle_Speed/1 -> VehBusCreat/18(IMAPve_g_SW_Angle_Speed)
  IMAPve_d_BCM_BrakeLamp_State/1 -> VehBusCreat/53(IMAPve_d_BCM_BrakeLamp_State)
  IMAPve_g_R0_C3/1 -> FusionBusCreat/54(IMAPve_g_R0_C3)
  IMAPve_d_R0_Q/1 -> FusionBusCreat/56(IMAPve_d_R0_Q)
  IMAPve_d_EPB_Status/1 -> VehBusCreat/56(IMAPve_d_EPB_Status)
  IMAPve_d_R0_Type/1 -> FusionBusCreat/57(IMAPve_d_R0_Type)
  IMAPve_d_L0_LC/1 -> FusionBusCreat/50(IMAPve_d_L0_LC)
  IMAPve_g_R0_C1/1 -> FusionBusCreat/52(IMAPve_g_R0_C1)
  IMAPva_d_obj_JA/1 -> FusionBusCreat/36(IMAPva_d_obj_JA)
  IMAPve_g_R0_C0/1 -> FusionBusCreat/51(IMAPve_g_R0_C0)
  IMAPve_g_L0_TLC/1 -> FusionBusCreat/49(IMAPve_g_L0_TLC)
  IMAPve_d_Brake_Pedal_Fault/1 -> VehBusCreat/40(IMAPve_d_Brake_Pedal_Fault)
  IMAPve_d_L0_Type/1 -> FusionBusCreat/46(IMAPve_d_L0_Type)
  IMAPva_d_obj_MotionStatus/1 -> FusionBusCreat/33(IMAPva_d_obj_MotionStatus)
  IMAPve_g_L0_VR/1 -> FusionBusCreat/44(IMAPve_g_L0_VR)
  IMAPve_d_ACU_Driver_Belt/1 -> VehBusCreat/31(IMAPve_d_ACU_Driver_Belt)
  IMAPva_d_obj_TurnLight/1 -> FusionBusCreat/31(IMAPva_d_obj_TurnLight)
  IMAPve_d_Sensor_Status/1 -> FusionBusCreat/1(IMAPve_d_Sensor_Status)
  IMAPva_g_obj_vel_y/1 -> FusionBusCreat/13(IMAPva_g_obj_vel_y)
  IMAPve_d_EMS_Brake_Pedal/1 -> VehBusCreat/55(IMAPve_d_EMS_Brake_Pedal)
  IMAPve_g_SW_Angle/1 -> VehBusCreat/17(IMAPve_g_SW_Angle)
  IMAPva_d_obj_fusion_type/1 -> FusionBusCreat/24(IMAPva_d_obj_fusion_type)
  IMAPve_d_ESC_Hold_State/1 -> VehBusCreat/58(IMAPve_d_ESC_Hold_State)
  IMAPve_d_LF_Radar_Status/1 -> FusionBusCreat/2(IMAPve_d_LF_Radar_Status)
  IMAPve_d_ESC_AlarmSig/1 -> VehBusCreat/35(IMAPve_d_ESC_AlarmSig)
  IMAPva_g_obj_length/1 -> FusionBusCreat/23(IMAPva_g_obj_length)
  IMAPva_g_obj_vel_var_xy/1 -> FusionBusCreat/21(IMAPva_g_obj_vel_var_xy)
  IMAPva_g_obj_pos_var_y/1 -> FusionBusCreat/17(IMAPva_g_obj_pos_var_y)
  IMAPve_d_ESC_Veh_Standstill/1 -> VehBusCreat/27(IMAPve_d_ESC_Veh_Standstill)
  IMAPva_g_obj_vel_var_x/1 -> FusionBusCreat/19(IMAPva_g_obj_vel_var_x)
  IMAPve_d_SWS_Fault_Code/1 -> VehBusCreat/32(IMAPve_d_SWS_Fault_Code)
  IMAPve_d_LR_Radar_Status/1 -> FusionBusCreat/4(IMAPve_d_LR_Radar_Status)
  IMAPve_d_Signal_Time_Stamp/1 -> VehBusCreat/60(IMAPve_d_Signal_Time_Stamp)
  IMAPve_d_SCC_Left_SwitchSig/1 -> VehBusCreat/23(IMAPve_d_SCC_Left_SwitchSig)
  IMAPva_g_obj_pos_x/1 -> FusionBusCreat/10(IMAPva_g_obj_pos_x)
  IMAPva_d_obj_AEB/1 -> FusionBusCreat/34(IMAPva_d_obj_AEB)
  IMAPve_d_ESC_RR_WheelPulVal/1 -> VehBusCreat/45(IMAPve_d_ESC_RR_WheelPulVal)
  IMAPva_g_obj_acc_y/1 -> FusionBusCreat/15(IMAPva_g_obj_acc_y)
  IMAPve_d_Fusion_Status/1 -> FusionBusCreat/6(IMAPve_d_Fusion_Status)
  IMAPva_g_obj_vel_x/1 -> FusionBusCreat/12(IMAPva_g_obj_vel_x)
  IMAPve_g_L0_W/1 -> FusionBusCreat/48(IMAPve_g_L0_W)
  IMAPve_d_RR_Radar_Status/1 -> FusionBusCreat/5(IMAPve_d_RR_Radar_Status)
  IMAPve_g_ESC_Brake_Press/1 -> VehBusCreat/13(IMAPve_g_ESC_Brake_Press)
  IMAPve_d_ESC_AEB_Available/1 -> VehBusCreat/49(IMAPve_d_ESC_AEB_Available)
  IMAPve_d_EMS_Engine_Status/1 -> VehBusCreat/47(IMAPve_d_EMS_Engine_Status)
  IMAPva_g_obj_age/1 -> FusionBusCreat/30(IMAPva_g_obj_age)
  IMAPva_g_obj_width/1 -> FusionBusCreat/22(IMAPva_g_obj_width)
  IMAPve_d_Radar_State/1 -> VehBusCreat/59(IMAPve_d_Radar_State)
  IMAPve_d_ESC_RL_WheelPulVal/1 -> VehBusCreat/44(IMAPve_d_ESC_RL_WheelPulVal)
  IMAPve_d_ESC_VehSpd_Valid/1 -> VehBusCreat/39(IMAPve_d_ESC_VehSpd_Valid)
  IMAPva_d_obj_class/1 -> FusionBusCreat/25(IMAPva_d_obj_class)
  IMAPve_d_ESC_ABS_Active/1 -> VehBusCreat/41(IMAPve_d_ESC_ABS_Active)
  IMAPve_d_ESC_TCS_Active/1 -> VehBusCreat/38(IMAPve_d_ESC_TCS_Active)
  IMAPva_d_obj_cam_asso_id/1 -> FusionBusCreat/28(IMAPva_d_obj_cam_asso_id)
  IMAPve_d_ESC_AEB_Status/1 -> VehBusCreat/48(IMAPve_d_ESC_AEB_Status)
  IMAPve_d_ESC_MSR_Active/1 -> VehBusCreat/37(IMAPve_d_ESC_MSR_Active)
  IMAPve_d_ESC_FR_WheelPulVal/1 -> VehBusCreat/43(IMAPve_d_ESC_FR_WheelPulVal)
  FDMMve_d_JaFcnConf/1 -> VehBusCreat/2(FDMMve_d_JaFcnConf)
  IMAPva_g_obj_acc_x/1 -> FusionBusCreat/14(IMAPva_g_obj_acc_x)
  IMAPva_d_obj_status/1 -> FusionBusCreat/27(IMAPva_d_obj_status)
  IMAPve_d_SWS_Failure_Status/1 -> VehBusCreat/33(IMAPve_d_SWS_Failure_Status)
  IMAPve_d_ESC_FL_WheelPulVal/1 -> VehBusCreat/42(IMAPve_d_ESC_FL_WheelPulVal)
  IMAPve_d_BCM_CHMSL_Status/1 -> VehBusCreat/52(IMAPve_d_BCM_CHMSL_Status)
  IMAPve_d_ESC_OFF/1 -> VehBusCreat/34(IMAPve_d_ESC_OFF)
  IMAPva_g_obj_pos_var_x/1 -> FusionBusCreat/16(IMAPva_g_obj_pos_var_x)
  IMAPve_d_BCM_FrontWiper_State/1 -> VehBusCreat/51(IMAPve_d_BCM_FrontWiper_State)
  IMAPve_d_Lane_Valid/1 -> FusionBusCreat/37(IMAPve_d_Lane_Valid)
  IMAPve_d_BCM_Left_Light/1 -> VehBusCreat/20(IMAPve_d_BCM_Left_Light)
  IMAPve_d_TCU_Target_Gear/1 -> VehBusCreat/29(IMAPve_d_TCU_Target_Gear)
  IMAPve_g_L0_C3/1 -> FusionBusCreat/43(IMAPve_g_L0_C3)
  IMAPve_d_BCM_Opening_State/1 -> VehBusCreat/22(IMAPve_d_BCM_Opening_State)
  IMAPve_d_TCU_AT_Failure/1 -> VehBusCreat/46(IMAPve_d_TCU_AT_Failure)
  IMAPve_g_ESC_Static_Slope/1 -> VehBusCreat/14(IMAPve_g_ESC_Static_Slope)
  IMAPve_d_BCM_Ignition_State/1 -> VehBusCreat/30(IMAPve_d_BCM_Ignition_State)
  IMAPve_g_EMS_RealPedal/1 -> VehBusCreat/25(IMAPve_g_EMS_RealPedal)
  IMAPve_d_ESC_ESC_Active/1 -> VehBusCreat/36(IMAPve_d_ESC_ESC_Active)
  IMAPve_d_SCC_Right_SwitchSig/1 -> VehBusCreat/24(IMAPve_d_SCC_Right_SwitchSig)
  IMAPve_d_EPS_Error_State/1 -> VehBusCreat/5(IMAPve_d_EPS_Error_State)
  IMAPve_d_BCM_Right_Light/1 -> VehBusCreat/21(IMAPve_d_BCM_Right_Light)
  IMAPve_g_ESC_DySlope_Accuracy/1 -> VehBusCreat/15(IMAPve_g_ESC_DySlope_Accuracy)
  IMAPve_g_EMS_ACC_VirtualPedal/1 -> VehBusCreat/26(IMAPve_g_EMS_ACC_VirtualPedal)
  IMAPve_d_ACU_Passenger_Belt/1 -> VehBusCreat/54(IMAPve_d_ACU_Passenger_Belt)
  IMAPva_d_obj_lane/1 -> FusionBusCreat/26(IMAPva_d_obj_lane)
  IMAPve_g_ESC_LatAcc/1 -> VehBusCreat/6(IMAPve_g_ESC_LatAcc)
  IMAPve_d_ESC_LonAcc_Valid/1 -> VehBusCreat/12(IMAPve_d_ESC_LonAcc_Valid)
  IMAPva_g_obj_pos_var_xy/1 -> FusionBusCreat/18(IMAPva_g_obj_pos_var_xy)
  IMAPve_g_ESC_DySlope/1 -> VehBusCreat/16(IMAPve_g_ESC_DySlope)
  IMAPva_g_obj_con/1 -> FusionBusCreat/29(IMAPva_g_obj_con)
  IMAPve_g_ESC_YawRate/1 -> VehBusCreat/7(IMAPve_g_ESC_YawRate)
  IMAPve_d_TCU_Actual_Gear/1 -> VehBusCreat/28(IMAPve_d_TCU_Actual_Gear)
  IMAPve_g_R0_W/1 -> FusionBusCreat/59(IMAPve_g_R0_W)
  IMAPve_g_EPS_SW_Trq/1 -> VehBusCreat/4(IMAPve_g_EPS_SW_Trq)
  IMAPve_g_ESC_VehSpd/1 -> VehBusCreat/10(IMAPve_g_ESC_VehSpd)
  JABSve_d_DecelReq_2/1 -> JABSve_d_Switching/1

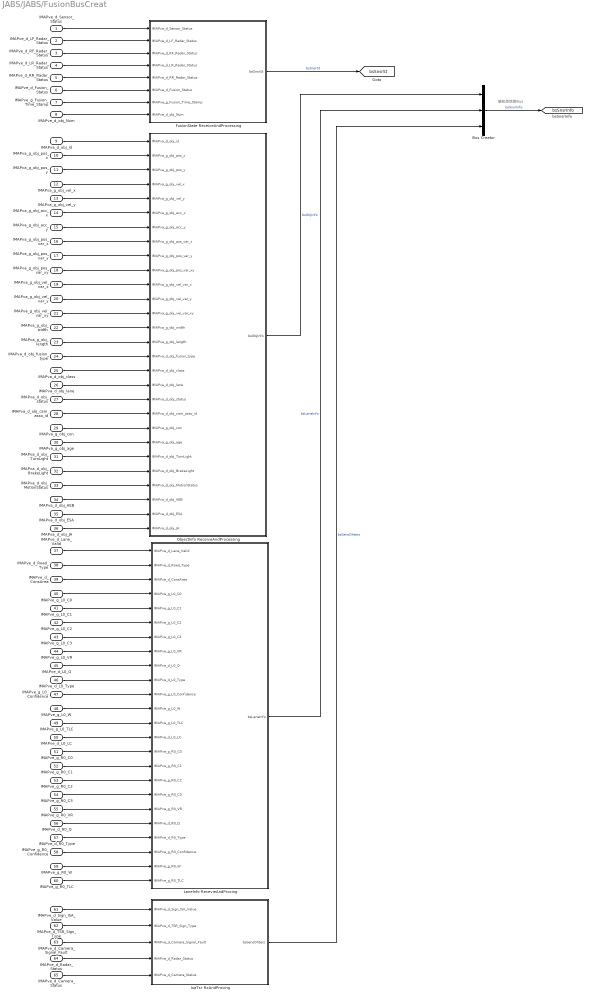
== system JABS/JABS/FusionBusCreat ==
  note: 感知类信息Bus
  IMAPve_d_Sensor_Status : Inport
  IMAPve_d_LF_Radar_Status : Inport  Port=2
  IMAPve_d_RF_Radar_Status : Inport  Port=3
  IMAPve_d_LR_Radar_Status : Inport  Port=4
  IMAPve_d_RR_Radar_Status : Inport  Port=5
  IMAPve_d_Fusion_Status : Inport  Port=6
  IMAPve_g_Fusion_Time_Stamp : Inport  Port=7
  IMAPve_d_obj_Num : Inport  Port=8
  IMAPva_d_obj_id : Inport  Port=9
  IMAPva_g_obj_pos_x : Inport  Port=10
  IMAPva_g_obj_pos_y : Inport  Port=11
  IMAPva_g_obj_vel_x : Inport  Port=12
  IMAPva_g_obj_vel_y : Inport  Port=13
  IMAPva_g_obj_acc_x : Inport  Port=14
  IMAPva_g_obj_acc_y : Inport  Port=15
  IMAPva_g_obj_pos_var_x : Inport  Port=16
  IMAPva_g_obj_pos_var_y : Inport  Port=17
  IMAPva_g_obj_pos_var_xy : Inport  Port=18
  IMAPva_g_obj_vel_var_x : Inport  Port=19
  IMAPva_g_obj_vel_var_y : Inport  Port=20
  IMAPva_g_obj_vel_var_xy : Inport  Port=21
  IMAPva_g_obj_width : Inport  Port=22
  IMAPva_g_obj_length : Inport  Port=23
  IMAPva_d_obj_fusion_type : Inport  Port=24
  IMAPva_d_obj_class : Inport  Port=25
  IMAPva_d_obj_lane : Inport  Port=26
  IMAPva_d_obj_status : Inport  Port=27
  IMAPva_d_obj_cam_asso_id : Inport  Port=28
  IMAPva_g_obj_con : Inport  Port=29
  IMAPva_g_obj_age : Inport  Port=30
  IMAPva_d_obj_TurnLight : Inport  Port=31
  IMAPva_d_obj_BrakeLight : Inport  Port=32
  IMAPva_d_obj_MotionStatus : Inport  Port=33
  IMAPva_d_obj_AEB : Inport  Port=34
  IMAPva_d_obj_ESA : Inport  Port=35
  IMAPva_d_obj_JA : Inport  Port=36
  IMAPve_d_Lane_Valid : Inport  Port=37
  IMAPve_d_Road_Type : Inport  Port=38
  IMAPve_d_ConsArea : Inport  Port=39
  IMAPve_g_L0_C0 : Inport  Port=40
  IMAPve_g_L0_C1 : Inport  Port=41
  IMAPve_g_L0_C2 : Inport  Port=42
  IMAPve_g_L0_C3 : Inport  Port=43
  IMAPve_g_L0_VR : Inport  Port=44
  IMAPve_d_L0_Q : Inport  Port=45
  IMAPve_d_L0_Type : Inport  Port=46
  IMAPve_g_L0_Confidence : Inport  Port=47
  IMAPve_g_L0_W : Inport  Port=48
  IMAPve_g_L0_TLC : Inport  Port=49
  IMAPve_d_L0_LC : Inport  Port=50
  IMAPve_g_R0_C0 : Inport  Port=51
  IMAPve_g_R0_C1 : Inport  Port=52
  IMAPve_g_R0_C2 : Inport  Port=53
  IMAPve_g_R0_C3 : Inport  Port=54
  IMAPve_g_R0_VR : Inport  Port=55
  IMAPve_d_R0_Q : Inport  Port=56
  IMAPve_d_R0_Type : Inport  Port=57
  IMAPve_g_R0_Confidence : Inport  Port=58
  IMAPve_g_R0_W : Inport  Port=59
  IMAPve_g_R0_TLC : Inport  Port=60
  IMAPve_d_Sign_ISA_Value : Inport  Port=61
  IMAPve_d_TSR_Sign_Type : Inport  Port=62
  IMAPve_d_Camera_Signal_Fault : Inport  Port=63
  IMAPve_d_Radar_Status : Inport  Port=64
  IMAPve_d_Camera_Status : Inport  Port=65
  Bus Creator : BusCreator  Inputs=3
  FusionState ReceiveAndProcessing : Subsystem
  IsaTsr RxAndProcing : Subsystem
  LaneInfo RecevieAndProcing : Subsystem
  ObjectInfo ReceiveAndProcessing : Subsystem
  tag scope: bsSnsrInfo=global, bsSnsrSt=global
  wires:
  ObjectInfo ReceiveAndProcessing/1(bsObjInfo) -> Bus Creator/1  "bsObjInfo"
  IsaTsr RxAndProcing/1(bsSensOhters) -> Bus Creator/3  "bsSensOhters"
  LaneInfo RecevieAndProcing/1(bsLaneInfo) -> Bus Creator/2  "bsLaneInfo"
  FusionState ReceiveAndProcessing/1(bsSnsrSt) -> [bsSnsrSt]  "bsSnsrSt"
  IMAPve_d_RR_Radar_Status/1 -> FusionState ReceiveAndProcessing/5(IMAPve_d_RR_Radar_Status)
  IMAPve_d_LR_Radar_Status/1 -> FusionState ReceiveAndProcessing/4(IMAPve_d_LR_Radar_Status)
  IMAPve_d_Fusion_Status/1 -> FusionState ReceiveAndProcessing/6(IMAPve_d_Fusion_Status)
  IMAPve_g_Fusion_Time_Stamp/1 -> FusionState ReceiveAndProcessing/7(IMAPve_g_Fusion_Time_Stamp)
  IMAPve_d_RF_Radar_Status/1 -> FusionState ReceiveAndProcessing/3(IMAPve_d_RF_Radar_Status)
  IMAPve_d_LF_Radar_Status/1 -> FusionState ReceiveAndProcessing/2(IMAPve_d_LF_Radar_Status)
  IMAPve_d_Sensor_Status/1 -> FusionState ReceiveAndProcessing/1(IMAPve_d_Sensor_Status)
  IMAPva_g_obj_vel_y/1 -> ObjectInfo ReceiveAndProcessing/5(IMAPva_g_obj_vel_y)
  IMAPva_g_obj_vel_x/1 -> ObjectInfo ReceiveAndProcessing/4(IMAPva_g_obj_vel_x)
  IMAPva_g_obj_acc_x/1 -> ObjectInfo ReceiveAndProcessing/6(IMAPva_g_obj_acc_x)
  IMAPva_g_obj_pos_y/1 -> ObjectInfo ReceiveAndProcessing/3(IMAPva_g_obj_pos_y)
  IMAPva_g_obj_acc_y/1 -> ObjectInfo ReceiveAndProcessing/7(IMAPva_g_obj_acc_y)
  IMAPva_g_obj_pos_x/1 -> ObjectInfo ReceiveAndProcessing/2(IMAPva_g_obj_pos_x)
  IMAPva_g_obj_pos_var_x/1 -> ObjectInfo ReceiveAndProcessing/8(IMAPva_g_obj_pos_var_x)
  IMAPva_d_obj_id/1 -> ObjectInfo ReceiveAndProcessing/1(IMAPva_d_obj_id)
  IMAPva_g_obj_pos_var_y/1 -> ObjectInfo ReceiveAndProcessing/9(IMAPva_g_obj_pos_var_y)
  IMAPve_d_obj_Num/1 -> FusionState ReceiveAndProcessing/8(IMAPve_d_obj_Num)
  IMAPva_g_obj_pos_var_xy/1 -> ObjectInfo ReceiveAndProcessing/10(IMAPva_g_obj_pos_var_xy)
  IMAPva_g_obj_vel_var_x/1 -> ObjectInfo ReceiveAndProcessing/11(IMAPva_g_obj_vel_var_x)
  IMAPva_g_obj_vel_var_y/1 -> ObjectInfo ReceiveAndProcessing/12(IMAPva_g_obj_vel_var_y)
  IMAPva_g_obj_vel_var_xy/1 -> ObjectInfo ReceiveAndProcessing/13(IMAPva_g_obj_vel_var_xy)
  IMAPva_g_obj_width/1 -> ObjectInfo ReceiveAndProcessing/14(IMAPva_g_obj_width)
  IMAPva_g_obj_length/1 -> ObjectInfo ReceiveAndProcessing/15(IMAPva_g_obj_length)
  IMAPva_d_obj_fusion_type/1 -> ObjectInfo ReceiveAndProcessing/16(IMAPva_d_obj_fusion_type)
  IMAPva_d_obj_class/1 -> ObjectInfo ReceiveAndProcessing/17(IMAPva_d_obj_class)
  IMAPva_d_obj_lane/1 -> ObjectInfo ReceiveAndProcessing/18(IMAPva_d_obj_lane)
  IMAPva_d_obj_status/1 -> ObjectInfo ReceiveAndProcessing/19(IMAPva_d_obj_status)
  IMAPva_d_obj_cam_asso_id/1 -> ObjectInfo ReceiveAndProcessing/20(IMAPva_d_obj_cam_asso_id)
  IMAPva_g_obj_con/1 -> ObjectInfo ReceiveAndProcessing/21(IMAPva_g_obj_con)
  IMAPva_g_obj_age/1 -> ObjectInfo ReceiveAndProcessing/22(IMAPva_g_obj_age)
  IMAPva_d_obj_TurnLight/1 -> ObjectInfo ReceiveAndProcessing/23(IMAPva_d_obj_TurnLight)
  IMAPva_d_obj_BrakeLight/1 -> ObjectInfo ReceiveAndProcessing/24(IMAPva_d_obj_BrakeLight)
  IMAPva_d_obj_MotionStatus/1 -> ObjectInfo ReceiveAndProcessing/25(IMAPva_d_obj_MotionStatus)
  IMAPva_d_obj_AEB/1 -> ObjectInfo ReceiveAndProcessing/26(IMAPva_d_obj_AEB)
  IMAPva_d_obj_ESA/1 -> ObjectInfo ReceiveAndProcessing/27(IMAPva_d_obj_ESA)
  IMAPva_d_obj_JA/1 -> ObjectInfo ReceiveAndProcessing/28(IMAPva_d_obj_JA)
  IMAPve_g_L0_TLC/1 -> LaneInfo RecevieAndProcing/13(IMAPve_g_L0_TLC)
  IMAPve_g_L0_W/1 -> LaneInfo RecevieAndProcing/12(IMAPve_g_L0_W)
  IMAPve_d_L0_LC/1 -> LaneInfo RecevieAndProcing/14(IMAPve_d_L0_LC)
  IMAPve_g_L0_Confidence/1 -> LaneInfo RecevieAndProcing/11(IMAPve_g_L0_Confidence)
  IMAPve_g_R0_C0/1 -> LaneInfo RecevieAndProcing/15(IMAPve_g_R0_C0)
  IMAPve_d_L0_Type/1 -> LaneInfo RecevieAndProcing/10(IMAPve_d_L0_Type)
  IMAPve_g_R0_C1/1 -> LaneInfo RecevieAndProcing/16(IMAPve_g_R0_C1)
  IMAPve_g_R0_C2/1 -> LaneInfo RecevieAndProcing/17(IMAPve_g_R0_C2)
  IMAPve_g_R0_C3/1 -> LaneInfo RecevieAndProcing/18(IMAPve_g_R0_C3)
  IMAPve_g_R0_VR/1 -> LaneInfo RecevieAndProcing/19(IMAPve_g_R0_VR)
  IMAPve_d_R0_Q/1 -> LaneInfo RecevieAndProcing/20(IMAPve_d_R0_Q)
  IMAPve_d_L0_Q/1 -> LaneInfo RecevieAndProcing/9(IMAPve_d_L0_Q)
  IMAPve_d_R0_Type/1 -> LaneInfo RecevieAndProcing/21(IMAPve_d_R0_Type)
  IMAPve_g_L0_VR/1 -> LaneInfo RecevieAndProcing/8(IMAPve_g_L0_VR)
  IMAPve_g_R0_Confidence/1 -> LaneInfo RecevieAndProcing/22(IMAPve_g_R0_Confidence)
  IMAPve_g_R0_W/1 -> LaneInfo RecevieAndProcing/23(IMAPve_g_R0_W)
  IMAPve_g_R0_TLC/1 -> LaneInfo RecevieAndProcing/24(IMAPve_g_R0_TLC)
  IMAPve_g_L0_C3/1 -> LaneInfo RecevieAndProcing/7(IMAPve_g_L0_C3)
  IMAPve_g_L0_C2/1 -> LaneInfo RecevieAndProcing/6(IMAPve_g_L0_C2)
  IMAPve_g_L0_C1/1 -> LaneInfo RecevieAndProcing/5(IMAPve_g_L0_C1)
  IMAPve_g_L0_C0/1 -> LaneInfo RecevieAndProcing/4(IMAPve_g_L0_C0)
  IMAPve_d_ConsArea/1 -> LaneInfo RecevieAndProcing/3(IMAPve_d_ConsArea)
  IMAPve_d_Road_Type/1 -> LaneInfo RecevieAndProcing/2(IMAPve_d_Road_Type)
  IMAPve_d_Lane_Valid/1 -> LaneInfo RecevieAndProcing/1(IMAPve_d_Lane_Valid)
  IMAPve_d_Camera_Status/1 -> IsaTsr RxAndProcing/5(IMAPve_d_Camera_Status)
  IMAPve_d_TSR_Sign_Type/1 -> IsaTsr RxAndProcing/2(IMAPve_d_TSR_Sign_Type)
  IMAPve_d_Radar_Status/1 -> IsaTsr RxAndProcing/4(IMAPve_d_Radar_Status)
  IMAPve_d_Camera_Signal_Fault/1 -> IsaTsr RxAndProcing/3(IMAPve_d_Camera_Signal_Fault)
  IMAPve_d_Sign_ISA_Value/1 -> IsaTsr RxAndProcing/1(IMAPve_d_Sign_ISA_Value)
  Bus Creator/1 -> [bsSnsrInfo]  "bsSnsrInfo"
